simulink model "model"  (R2021a)
settings: Solver=ode23s  StartTime=0.0  StopTime=121  RelTol=1e-3
settings Model: Creator=dnavalos  LastModifiedBy=dnavalos

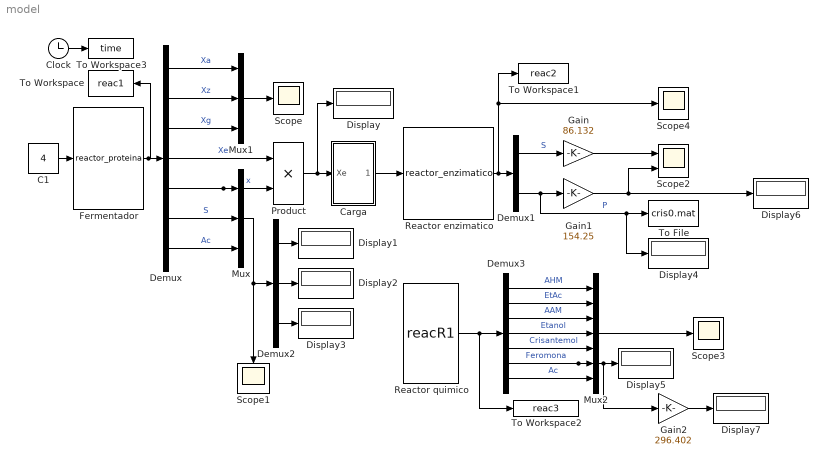
== system model ==
  C1 : Constant  Value=4
  Carga : Subsystem
  Clock : Clock
  Demux : Demux  Outputs=7
  Demux1 : Demux  Outputs=2
  Demux2 : Demux  Outputs=3
  Demux3 : Demux  Outputs=7
  Display{,1..7} (8 alike) : Display
  Fermentador : S-Function  FunctionName=reactor_proteina  SFunctionDeploymentMode=off  EnableBusSupport=off
      mask Display: image('reac.png'); % Use "Edit Image" on toolstrip to change.
  Gain : Gain  Gain=86.132
  Gain1 : Gain  Gain=154.25
  Gain2 : Gain  Gain=296.402
  Mux : Mux  Inputs=3
  Mux1 : Mux  Inputs=3
  Mux2 : Mux  Inputs=7
  Product : Product
  Reactor enzimatico : S-Function  FunctionName=reactor_enzimatico  SFunctionDeploymentMode=off  EnableBusSupport=off
      mask Display: image('reac2.jpg'); % Use "Edit Image" on toolstrip to change.
  Reactor quimico : S-Function  FunctionName=reacR1  SFunctionDeploymentMode=off  EnableBusSupport=off
      mask Display: image('reac3.jpeg'); % Use "Edit Image" on toolstrip to change.
  Scope{,1,3..4} (4 alike) : Scope
  Scope2 : Scope  NumInputPorts=2
  To File : ToFile  Filename=cris0.mat
  To Workspace : ToWorkspace  VariableName=reac1  SampleTime=-1
  To Workspace1 : ToWorkspace  VariableName=reac2  SampleTime=-1
  To Workspace2 : ToWorkspace  VariableName=reac3  SampleTime=-1
  To Workspace3 : ToWorkspace  VariableName=time  SampleTime=-1
  wires:
  C1/1 -> Fermentador/1
  Fermentador/1 -> To Workspace/1, Demux/1
  Demux/1 -> Mux1/1  "Xa"
  Demux/2 -> Mux1/2  "Xz"
  Demux/5 -> Product/2, Mux/1  "x"
  Demux/6 -> Mux/2  "S"
  Demux/7 -> Mux/3  "Ac"
  Mux/1 -> Demux2/1, Scope1/1
  Demux/3 -> Mux1/3  "Xg"
  Mux1/1 -> Scope/1
  Reactor enzimatico/1 -> Scope4/1, To Workspace1/1, Demux1/1
  Demux2/2 -> Display2/1
  Demux2/1 -> Display1/1
  Demux2/3 -> Display3/1
  Product/1 -> Carga/1(Xe), Display/1
  Demux/4 -> Product/1  "Xe"
  Carga/1(Out1) -> Reactor enzimatico/1
  Demux1/1 -> Gain/1  "S"
  Gain/1 -> Scope2/1
  Gain1/1 -> Scope2/2, Display6/1
  Demux1/2 -> Display4/1, To File/1, Gain1/1  "P"
  Reactor quimico/1 -> Demux3/1, To Workspace2/1
  Demux3/1 -> Mux2/1  "AHM"
  Demux3/2 -> Mux2/2  "EtAc"
  Demux3/3 -> Mux2/3  "AAM"
  Demux3/4 -> Mux2/4  "Etanol"
  Demux3/5 -> Mux2/5  "Crisantemol"
  Demux3/6 -> Gain2/1, Display5/1, Mux2/6  "Feromona"
  Mux2/1 -> Scope3/1
  Demux3/7 -> Mux2/7  "Ac"
  Clock/1 -> To Workspace3/1
  Gain2/1 -> Display7/1

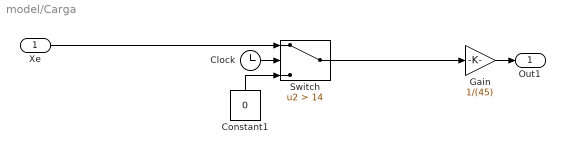
== system model/Carga ==
  Xe : Inport
  Clock : Clock
  Constant1 : Constant  Value=0
  Gain : Gain  Gain=1/(45)
  Switch : Switch  Criteria=u2 > Threshold  Threshold=14
  Out1 : Outport
  wires:
  Clock/1 -> Switch/2
  Constant1/1 -> Switch/3
  Xe/1 -> Switch/1
  Switch/1 -> Gain/1
  Gain/1 -> Out1/1
